simulink subsystem "dyn_model"  (R2023b)
settings: Solver=VariableStepAuto  StartTime=0.0  StopTime=10.0  RelTol=1e-3
model mask{Environment=0, Spacecraft=0, sc_type=0}
  mask prompts: Spacecraft "Spacecraft data"; sc_type "Spacecraft type (main/beacon)"
undefined symbols (not defined in the file or in its folder): srp, thrust
libraries: dyn_lib x3, sensors_subsystems x2, matrix_library x2, vrlib x2, sharedtransform x1
settings Model: Creator=brent  LastModifiedBy=brent

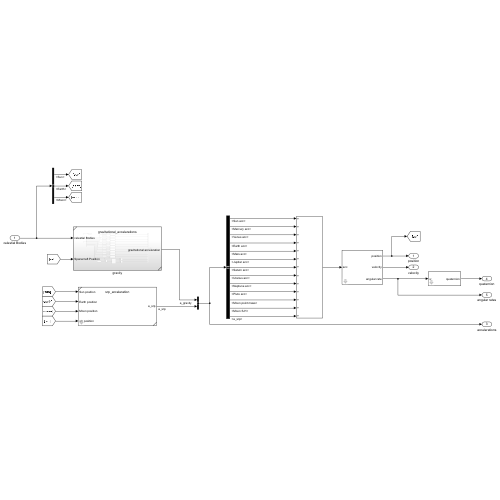
[thumbnail: Simulink's stored preview of the top-level diagram]
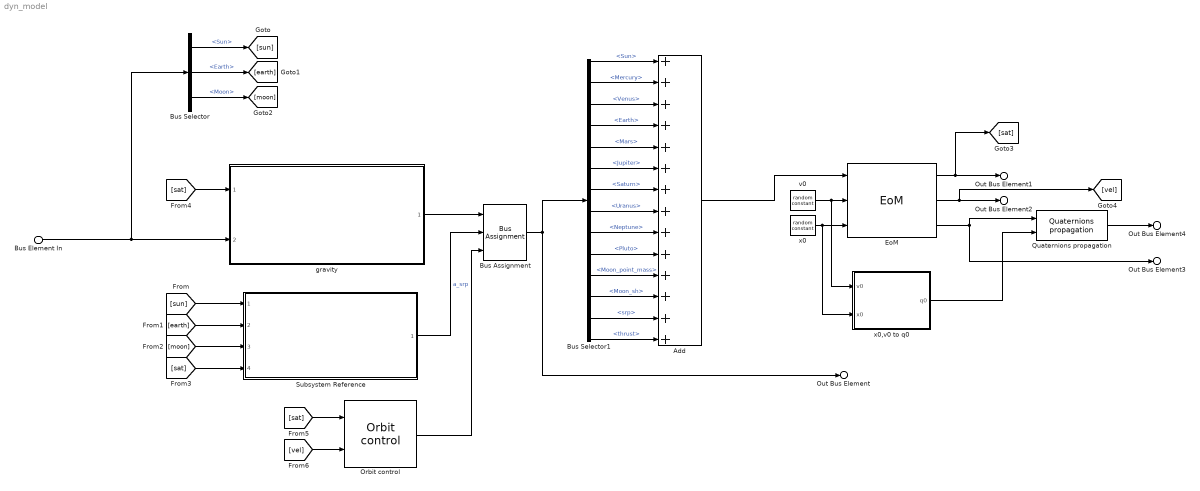
== system dyn_model ==
  Bus Element In : Inport  PortName=celestialBodies
  Add : Sum  Inputs=++++++++++++++
  Bus Assignment : BusAssignment  AssignedSignals=srp,thrust
  Bus Selector : BusSelector  OutputSignals=Sun,Earth,Moon
  Bus Selector1 : BusSelector  OutputSignals=Sun,Mercury,Venus,Earth,Mars,Jupiter,Saturn,Uranus,Neptune,Pluto,Moon_point_mass,Moon_sh,srp,thrust
  EoM : dyn_lib/EoM
      settings: SourceProductName=Dynamics library
  Orbit control : dyn_lib/Orbit control  VariantControl=Subsystem  flag=sc_type
      settings: SourceProductName=Dynamics library
  Quaternions propagation : dyn_lib/Quaternions propagation
      settings: SourceProductName=Dynamics library
  Subsystem Reference : Subsystem  ReferencedSubsystem=srp_acceleration  earth_radius=Environment.Earth.radius.value  sun_radius=Environment.Sun.radius.value  moon_radius=Environment.Moon.radius.value  C_R=Spacecraft.rp_coeff.value  A_sc=Spacecraft.radius.value^2*pi  m_sc=Spacecraft.mass.value  AU=Environment.AU.value  P=Environment.Sun.P.value
  gravity : Subsystem  ReferencedSubsystem=gravitational_accelerations
  v0 : sensors_subsystems/random constant  mean=Spacecraft.v0.nominal  dev=Spacecraft.v0.std
      settings: SourceProductName=Sensors library
  x0 : sensors_subsystems/random constant  mean=Spacecraft.x0.nominal  dev=Spacecraft.x0.std
      settings: SourceProductName=Sensors library
  x0,v0 to q0 : Subsystem  TreatAsAtomicUnit=on  SystemSampleTime=1e8
  Out Bus Element1 : Outport  PortName=spacecraftState  Element=x
  Out Bus Element2 : Outport  PortName=spacecraftState  Element=v
  Out Bus Element3 : Outport  PortName=spacecraftState  Element=w
  Out Bus Element4 : Outport  PortName=spacecraftState  Element=q
  Out Bus Element : Outport  PortName=spacecraftState  Element=a
  wires:
  [sat] -> gravity/1
  Bus Element In/1 -> Bus Selector/1, gravity/2
  [earth] -> Subsystem Reference/2
  [moon] -> Subsystem Reference/3
  EoM/3 -> Quaternions propagation/1, Out Bus Element3/1
  [sat] -> Subsystem Reference/4
  Bus Selector/3 -> [moon]  "<Moon>"
  EoM/2 -> Out Bus Element2/1, [vel]
  Quaternions propagation/1 -> Out Bus Element4/1
  [sun] -> Subsystem Reference/1
  Bus Selector/1 -> [sun]  "<Sun>"
  Bus Selector/2 -> [earth]  "<Earth>"
  Subsystem Reference/1 -> Bus Assignment/2  "a_srp"
  gravity/1 -> Bus Assignment/1
  Bus Assignment/1 -> Out Bus Element/1, Bus Selector1/1
  Bus Selector1/1 -> Add/1  "<Sun>"
  Bus Selector1/2 -> Add/2  "<Mercury>"
  Bus Selector1/3 -> Add/3  "<Venus>"
  Bus Selector1/4 -> Add/4  "<Earth>"
  Bus Selector1/5 -> Add/5  "<Mars>"
  Bus Selector1/6 -> Add/6  "<Jupiter>"
  Bus Selector1/7 -> Add/7  "<Saturn>"
  Bus Selector1/8 -> Add/8  "<Uranus>"
  Bus Selector1/9 -> Add/9  "<Neptune>"
  Bus Selector1/10 -> Add/10  "<Pluto>"
  Bus Selector1/11 -> Add/11  "<Moon_point_mass>"
  Bus Selector1/12 -> Add/12  "<Moon_sh>"
  Bus Selector1/13 -> Add/13  "<srp>"
  Add/1 -> EoM/1
  EoM/1 -> [sat], Out Bus Element1/1
  Bus Selector1/14 -> Add/14  "<thrust>"
  Orbit control/1 -> Bus Assignment/3
  [sat] -> Orbit control/1
  [vel] -> Orbit control/2
  x0/1 -> EoM/3, x0,v0 to q0/2(x0)
  v0/1 -> EoM/2, x0,v0 to q0/1(v0)
  x0,v0 to q0/1(q0) -> Quaternions propagation/2

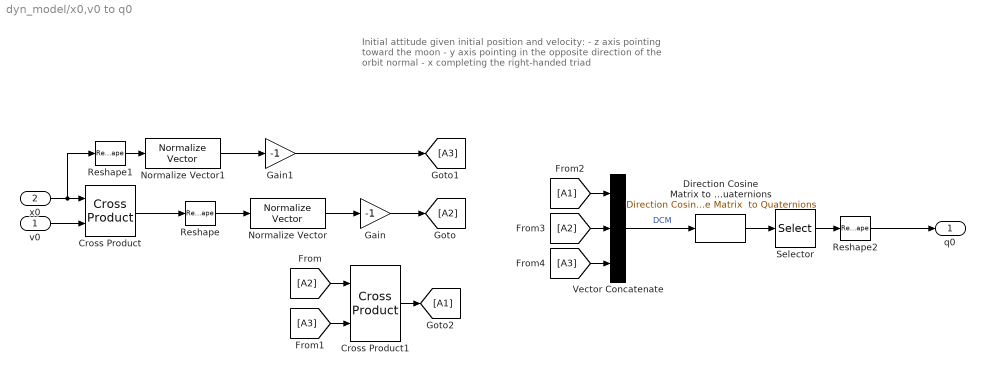
== system dyn_model/x0,v0 to q0 ==
  note: Initial attitude given initial position and velocity:
      | - z axis pointing toward the moon
      | - y axis pointing in the opposite direction of the orbit normal
      | - x completing the right-handed triad
  v0 : Inport
  x0 : Inport  Port=2
  Cross Product : matrix_library/Cross Product
  Cross Product1 : matrix_library/Cross Product
  Direction Cosine Matrix to Quaternions : sharedtransform/Direction Cosine Matrix  to Quaternions  aMode=0  action=None  tolerance=eps(2)
      settings: LibrarySourceBlock=|
      | aerolibtransform2/Direction Cosine Matrix
      | to Quaternions
  Gain : Gain  Gain=-1
  Gain1 : Gain  Gain=-1
  Normalize Vector : vrlib/Utilities/Normalize Vector  maxzero=0
  Normalize Vector1 : vrlib/Utilities/Normalize Vector  maxzero=0
  Reshape : Reshape  OutputDimensionality=Row vector (2-D)
  Reshape1 : Reshape  OutputDimensionality=Row vector (2-D)
  Reshape2 : Reshape  OutputDimensionality=Column vector (2-D)
  Selector : Selector  InputPortWidth=4  IndexOptions=Index vector (dialog)  Indices=[2 3 4 1]  OutputSizes=1
  Vector Concatenate : Concatenate  NumInputs=3  Mode=Multidimensional array
  q0 : Outport
  wires:
  Reshape2/1 -> q0/1
  Selector/1 -> Reshape2/1
  Direction Cosine Matrix to Quaternions/1 -> Selector/1
  Vector Concatenate/1 -> Direction Cosine Matrix to Quaternions/1  "DCM"
  [A3] -> Vector Concatenate/3
  [A2] -> Vector Concatenate/2
  [A1] -> Vector Concatenate/1
  Cross Product1/1 -> [A1]
  [A3] -> Cross Product1/2
  [A2] -> Cross Product1/1
  Gain1/1 -> [A3]
  Normalize Vector1/1 -> Gain1/1
  Reshape1/1 -> Normalize Vector1/1
  Gain/1 -> [A2]
  Normalize Vector/1 -> Gain/1
  Reshape/1 -> Normalize Vector/1
  Cross Product/1 -> Reshape/1
  v0/1 -> Cross Product/2
  x0/1 -> Cross Product/1, Reshape1/1
